simulink model "test_constantPump"  (R2013a)
settings: Solver=ode15s  StartTime=0.0  StopTime=3  RelTol=1e-3
libraries: fl_lib x7, nesl_utility x5, usask_hyd_ssc_lib x1
settings Model: Creator=tkw954  LastModifiedBy=tkw954
settings SimscapeCC: SimscapeLogType=all

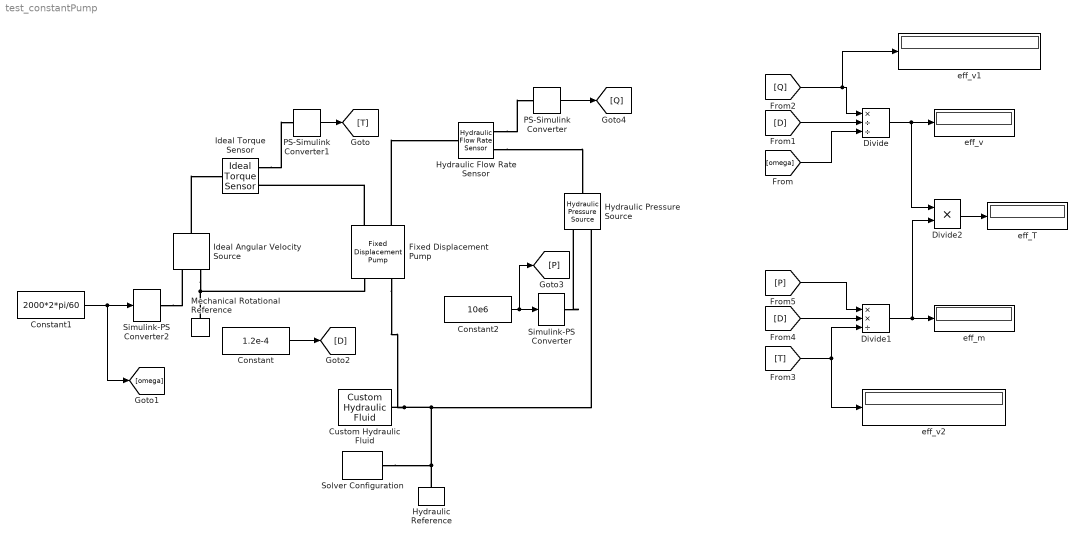
== system test_constantPump ==
  Constant : Constant  Value=1.2e-4
  Constant1 : Constant  Value=2000*2*pi/60
  Constant2 : Constant  Value=10e6
  Custom Hydraulic Fluid : fl_lib/Hydraulic/Hydraulic Utilities/Custom Hydraulic Fluid  density=850 kg/m^3  viscosity_kin=40e-3/850 m^2/s  bulk=0.8e9 Pa  alpha=0.005  LocalVarLogging=[]
  Divide : Product  Inputs=*//
  Divide1 : Product  Inputs=**/
  Divide2 : Product  Inputs=**
  Fixed Displacement Pump : usask_hyd_ssc_lib/Fixed Displacement Pump  D=1.2e-4 m^3/rad  eff_v0=0.9  eff_m0=0.9  p0=10e6 Pa  omega0=2000 rpm  mu0=40e-3 s*Pa  Cs=0  CD=0  mu=40e-3 s*Pa  density=860 kg/m^3  t_Log=off  q_Log=off  p_Log=off  omega_Log=off  LocalVarNames=|t|q|p|omega  LocalVarDescs=|torque|flow|Pressure|shaft speed  LocalVarLogging=[0 0 0 0]
  Hydraulic Flow Rate Sensor : fl_lib/Hydraulic/Hydraulic Sensors/Hydraulic Flow Rate Sensor  q_Log=off  p_Log=off  LocalVarNames=|q|p  LocalVarDescs=|q|p  LocalVarLogging=[0 0]
  Hydraulic Pressure Source : fl_lib/Hydraulic/Hydraulic Sources/Hydraulic Pressure Source  q_Log=off  p_Log=off  LocalVarNames=|q|p  LocalVarDescs=|q|p  LocalVarLogging=[0 0]
  Hydraulic Reference : fl_lib/Hydraulic/Hydraulic Elements/Hydraulic Reference  q_Log=off  LocalVarNames=|q  LocalVarDescs=|q  LocalVarLogging=0
  Ideal Angular Velocity Source : fl_lib/Mechanical/Mechanical Sources/Ideal Angular Velocity Source  w_Log=off  t_Log=off  LocalVarNames=|w|t  LocalVarDescs=|w|t  LocalVarLogging=[0 0]
  Ideal Torque Sensor : fl_lib/Mechanical/Mechanical Sensors/Ideal Torque Sensor  w_Log=off  t_Log=off  LocalVarNames=|w|t  LocalVarDescs=|w|t  LocalVarLogging=[0 0]
  Mechanical Rotational Reference : fl_lib/Mechanical/Rotational Elements/Mechanical Rotational Reference  t_Log=off  LocalVarNames=|t  LocalVarDescs=|t  LocalVarLogging=0
  PS-Simulink Converter : nesl_utility/PS-Simulink Converter  PhysicalDomain=network_engine_domain  SubClassName=ps_output  LeftPortType=input  RightPortType=output  PseudoPeriodic=off  Frequencies=[]  Unit=1  AffineConversion=off
  PS-Simulink Converter1 : nesl_utility/PS-Simulink Converter  PhysicalDomain=network_engine_domain  SubClassName=ps_output  LeftPortType=input  RightPortType=output  PseudoPeriodic=off  Frequencies=[]  Unit=1  AffineConversion=off
  Simulink-PS Converter : nesl_utility/Simulink-PS Converter  PhysicalDomain=network_engine_domain  SubClassName=ps_input  LeftPortType=input  RightPortType=output  PseudoPeriodic=off  Frequencies=[]  NoiseDistribution=none  NoiseParameters=[]  Unit=1  AffineConversion=off  InputFiltering=off  SimscapeFilterOrder=1  InputFilterTimeConstant=0.001  UdotUserProvided=1
  Simulink-PS Converter2 : nesl_utility/Simulink-PS Converter  PhysicalDomain=network_engine_domain  SubClassName=ps_input  LeftPortType=input  RightPortType=output  PseudoPeriodic=off  Frequencies=[]  NoiseDistribution=none  NoiseParameters=[]  Unit=rad/s  AffineConversion=off  InputFiltering=off  SimscapeFilterOrder=1  InputFilterTimeConstant=0.001  UdotUserProvided=1
  Solver Configuration : nesl_utility/Solver Configuration  PhysicalDomain=network_engine_domain  SubClassName=solver  LeftPortType=input  RightPortType=generic  Accelerate=off  Tones=[]  Harmonics=[]  SimulateNoise=off  Profile=off  UseLocalSampling=off  EnableSwitchedLinearOptims=on  FrequencyDomain=off  UseCCode=off  UseNewInitialization=off  DoDC=off  ResidualTolerance=1e-09  UseLocalSolver=off  LocalSolverChoice=NE_BACKWARD_EULER_ADVANCER  LocalSolverSampleTime=0.001  DoFixedCost=off  MaxNonlinIter=3  MaxModeIter=2  LinearAlgebra=Sparse  DelaysMemoryBudget=1024
  eff_T : Display
  eff_m : Display
  eff_v : Display
  eff_v1 : Display
  eff_v2 : Display
  wires:
  Constant/1 -> [D]
  Constant2/1 -> [P], Simulink-PS Converter/1
  PS-Simulink Converter1/1 -> [T]
  Constant1/1 -> [omega], Simulink-PS Converter2/1
  PS-Simulink Converter/1 -> [Q]
  [Q] -> eff_v1/1, Divide/1
  Divide/1 -> Divide2/1, eff_v/1
  Divide1/1 -> Divide2/2, eff_m/1
  [D] -> Divide/2
  [omega] -> Divide/3
  [P] -> Divide1/1
  [D] -> Divide1/2
  [T] -> Divide1/3, eff_v2/1
  Divide2/1 -> eff_T/1
  connections:
  Simulink-PS Converter/RConn1 -- Hydraulic Pressure Source/RConn1
  Fixed Displacement Pump/RConn2 -- Hydraulic Flow Rate Sensor/LConn1
  Hydraulic Flow Rate Sensor/RConn1 -- PS-Simulink Converter/LConn1
  Hydraulic Reference/LConn1 -- Solver Configuration/RConn1 -- Hydraulic Pressure Source/RConn2 -- Fixed Displacement Pump/LConn2 -- Custom Hydraulic Fluid/RConn1
  Hydraulic Flow Rate Sensor/RConn2 -- Hydraulic Pressure Source/LConn1
  Ideal Angular Velocity Source/LConn1 -- Ideal Torque Sensor/LConn1
  Fixed Displacement Pump/RConn1 -- Ideal Torque Sensor/RConn1
  Ideal Angular Velocity Source/RConn2 -- Fixed Displacement Pump/LConn1 -- Mechanical Rotational Reference/LConn1
  Simulink-PS Converter2/RConn1 -- Ideal Angular Velocity Source/RConn1
  Ideal Torque Sensor/RConn2 -- PS-Simulink Converter1/LConn1
